simulink model "dff3"  (Simulink 3.00)
settings: Solver=ode45  SolverMode=SingleTasking  StartTime=0.0  StopTime=20  MaxStep=.010  RelTol=1e-3  AbsTol=1e-3
settings Model: TimeSaveName=t  SaveOutput=off

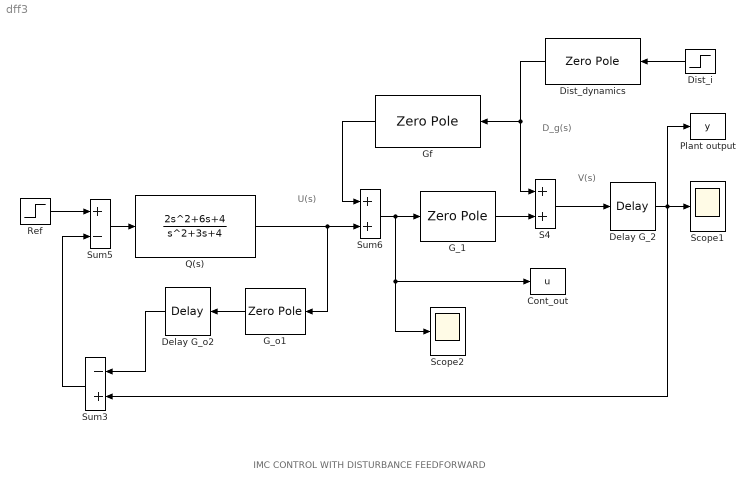
== system dff3 ==
  note: U(s)
  note: D_g(s)
  note: V(s)
  note: IMC CONTROL WITH DISTURBANCE FEEDFORWARD
  Cont_out : ToWorkspace  VariableName=u  SampleTime=0  SaveFormat=Matrix
      settings: Buffer=6000
  Delay G_2 : TransportDelay  DelayTime=2  InitialInput=0  BufferSize=4096
  Delay G_o2 : TransportDelay  Orientation=left  DelayTime=2.0  InitialInput=0  BufferSize=4096
  Dist_dynamics : ZeroPole  Orientation=left  Zeros=[]  Poles=[-3;-8]  Gain=[24]
  Dist_i : Step  Orientation=left  Time=10  Before=0  After=1  SampleTime=0
  G_1 : ZeroPole  Zeros=[]  Poles=[-1]  Gain=[1]
  G_o1 : ZeroPole  Orientation=left  Zeros=[]  Poles=[-1]  Gain=[1]
  Gf : ZeroPole  Orientation=left  Zeros=[-1]  Poles=[-10]  Gain=[-10]
  Plant output : ToWorkspace  VariableName=y  SampleTime=0  SaveFormat=Matrix
      settings: Buffer=6000
  Q(s) : TransferFcn  Numerator="[2  6 4]"  Denominator="[1  3 4]"
  Ref : Step  Time=1  Before=0  After=1  SampleTime=0
  S4 : Sum  Inputs=++  SaturateOnIntegerOverflow=on
  Scope1 : Scope
      settings: TickLabels=on  TimeRange=20.000000  YMin=-2.000000  YMax=2.000000  SaveToWorkspace=off  SaveName=ScopeData  DataFormat=Matrix
  Scope2 : Scope
      settings: TickLabels=on  TimeRange=20.000000  YMin=-4.000000  YMax=4.000000  SaveToWorkspace=off  SaveName=ScopeData  DataFormat=Matrix
  Sum3 : Sum  Orientation=left  Inputs=-+  SaturateOnIntegerOverflow=on
  Sum5 : Sum  Inputs=+-  SaturateOnIntegerOverflow=on
  Sum6 : Sum  Inputs=++  SaturateOnIntegerOverflow=on
  wires:
  S4/1 -> Delay G_2/1
  Delay G_2/1 -> Scope1/1, Plant output/1, Sum3/2
  G_o1/1 -> Delay G_o2/1
  Delay G_o2/1 -> Sum3/1
  Sum5/1 -> Q(s)/1
  Ref/1 -> Sum5/1
  Sum3/1 -> Sum5/2
  G_1/1 -> S4/2
  Gf/1 -> Sum6/1
  Sum6/1 -> G_1/1, Scope2/1, Cont_out/1
  Dist_i/1 -> Dist_dynamics/1
  Dist_dynamics/1 -> S4/1, Gf/1
  Q(s)/1 -> Sum6/2, G_o1/1
